simulink model "model3"  (R2014b)
settings: Solver=ode45  StartTime=0.0  StopTime=90  MaxStep=0.1  RelTol=1e-3
settings Model: Creator=Shane Reynolds  LastModifiedBy=Shane Reynolds

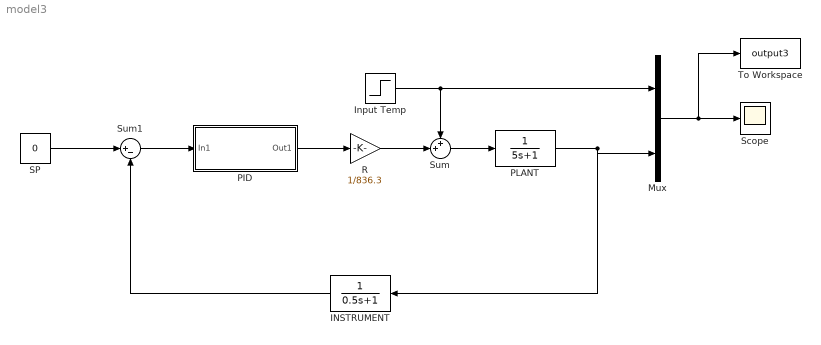
== system model3 ==
  INSTRUMENT : TransferFcn  Denominator=[0.5 1]
  Input Temp : Step  After=10  SampleTime=0
  Mux : Mux  Inputs=2
  PID : Subsystem
  PLANT : TransferFcn  Denominator=[5 1]
  R : Gain  Gain=1/836.3
  SP : Constant  Value=0
  Scope : Scope
  Sum : Sum  Inputs=++|
  Sum1 : Sum  Inputs=|+-
  To Workspace : ToWorkspace  VariableName=output3  SaveFormat=Timeseries  SampleTime=-1
  wires:
  R/1 -> Sum/2
  Sum/1 -> PLANT/1
  PLANT/1 -> INSTRUMENT/1, Mux/2
  Sum1/1 -> PID/1(In1)
  PID/1(Out1) -> R/1
  INSTRUMENT/1 -> Sum1/2
  SP/1 -> Sum1/1
  Mux/1 -> To Workspace/1, Scope/1
  Input Temp/1 -> Mux/1, Sum/1

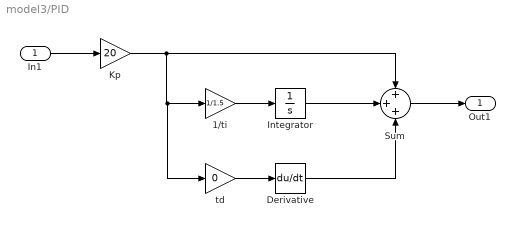
== system model3/PID ==
  In1 : Inport
  1/ti : Gain  Gain=1/1.5
  Derivative : Derivative
  Integrator : Integrator
  "Kp " : Gain  Gain=20
  Sum : Sum  Inputs=+++
  td : Gain  Gain=0
  Out1 : Outport
  wires:
  1/ti/1 -> Integrator/1
  td/1 -> Derivative/1
  Integrator/1 -> Sum/2
  Sum/1 -> Out1/1
  "Kp "/1 -> td/1, 1/ti/1, Sum/1
  In1/1 -> "Kp "/1
  Derivative/1 -> Sum/3
